simulink model "sim_PD_Control_wGC"  (R2020a)
settings: Solver=VariableStepAuto  StartTime=0.0  StopTime=T(end)  RelTol=1e-3
values from neighbouring files (symbols this model uses):
  q0 = zeros(1,NLinks)    [RobotPlot.m]
undefined symbols (not defined in the file or in its folder): B_accel, C_q, Fv_dq, fwdkin, G_q, Jadq, Jtrans, NLinks, T_step
settings Model: SimulationMode=accelerator  Creator=Dallas  LastModifiedBy=Dallas
settings DataIOCC: SaveFormat=Array  SaveOutput=off  SaveTime=off  ReturnWorkspaceOutputs=off

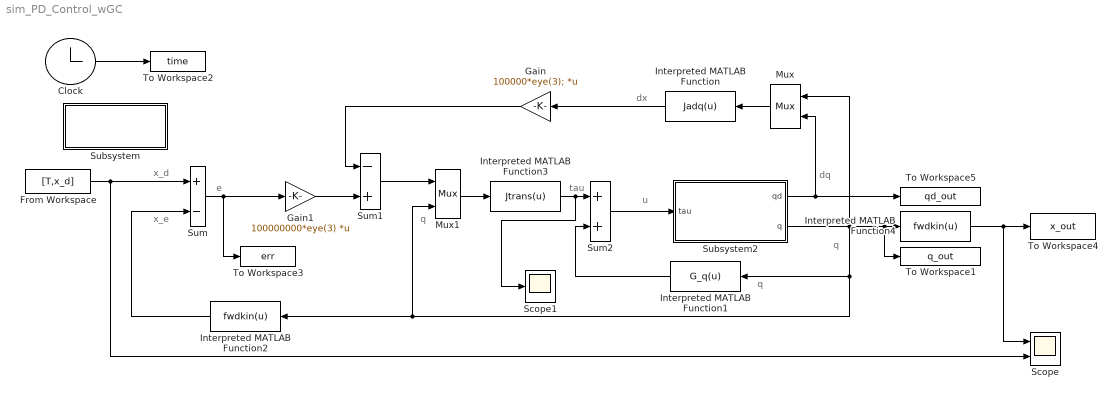
== system sim_PD_Control_wGC ==
  note: tau
  note: dx
  note: u
  note: q
  note: dq
  note: e
  note: x_e
  note: x_d
  note: q
  note: q
  Clock : Clock
  From Workspace : FromWorkspace  VariableName=[T,x_d]  SampleTime=T_step
  Gain : Gain  Gain=100000*eye(3);  Multiplication=Matrix(K*u)
      mask Display: disp('Kd')
  Gain1 : Gain  Gain=100000000*eye(3)  Multiplication=Matrix(K*u)
      mask Display: disp('Kp')
  Interpreted MATLAB Function : MATLABFcn  MATLABFcn=Jadq(u)  OutputDimensions=3
      mask Display: disp('Ja(q)*dq')
  Interpreted MATLAB Function1 : MATLABFcn  MATLABFcn=G_q(u)  OutputDimensions=NLinks
      mask Display: disp('G(q)')
  Interpreted MATLAB Function2 : MATLABFcn  MATLABFcn=fwdkin(u)  OutputDimensions=3
      mask Display: disp('Fwd Kin(q)')
  Interpreted MATLAB Function3 : MATLABFcn  MATLABFcn=Jtrans(u)  OutputDimensions=NLinks
      mask Display: disp('trans(Ja(dx))')
  Interpreted MATLAB Function4 : MATLABFcn  MATLABFcn=fwdkin(u)  OutputDimensions=3
      mask Display: disp('Fwd Kin(q)')
  Mux : Mux  Inputs=[NLinks,NLinks]
  Mux1 : Mux  Inputs=[3,NLinks]
  Scope : Scope  NumInputPorts=2
  Scope1 : Scope
  Subsystem : Subsystem  StartFcn=global NLinks DoF  StopFcn=SimPlotsPDG
      mask Display: disp('Plot')
  Subsystem2 : Subsystem
      mask Display: disp('inv(B(q))*(tau-tau'')')
  Sum : Sum  Inputs=+-
  Sum1 : Sum  Inputs=-+
  Sum2 : Sum
  To Workspace1 : ToWorkspace  VariableName=q_out  SampleTime=T_step
      settings: MaxDataPoints=4001
      mask Display: disp('q_out')
  To Workspace2 : ToWorkspace  VariableName=time  SampleTime=-1
      settings: MaxDataPoints=4001
      mask Display: disp('time')
  To Workspace3 : ToWorkspace  VariableName=err  SampleTime=T_step
      settings: MaxDataPoints=4001
      mask Display: disp('err')
  To Workspace4 : ToWorkspace  VariableName=x_out  SampleTime=T_step
      settings: MaxDataPoints=4001
      mask Display: disp('X_EEffector')
  To Workspace5 : ToWorkspace  VariableName=qd_out  SampleTime=T_step
      settings: MaxDataPoints=4001
      mask Display: disp('qd_out')
  wires:
  From Workspace/1 -> Scope/2, Sum/1
  Sum2/1 -> Subsystem2/1(tau)
  Subsystem2/1(qd) -> To Workspace5/1, Mux/2
  Subsystem2/2(q) -> To Workspace1/1, Interpreted MATLAB Function4/1, Mux1/2, Interpreted MATLAB Function2/1, Interpreted MATLAB Function1/1, Mux/1
  Interpreted MATLAB Function2/1 -> Sum/2
  Clock/1 -> To Workspace2/1
  Interpreted MATLAB Function1/1 -> Sum2/2
  Interpreted MATLAB Function3/1 -> Scope1/1, Sum2/1
  Mux/1 -> Interpreted MATLAB Function/1
  Mux1/1 -> Interpreted MATLAB Function3/1
  Interpreted MATLAB Function4/1 -> Scope/1, To Workspace4/1
  Sum/1 -> Gain1/1, To Workspace3/1
  Interpreted MATLAB Function/1 -> Gain/1
  Gain/1 -> Sum1/1
  Sum1/1 -> Mux1/1
  Gain1/1 -> Sum1/2

== system sim_PD_Control_wGC/Subsystem ==

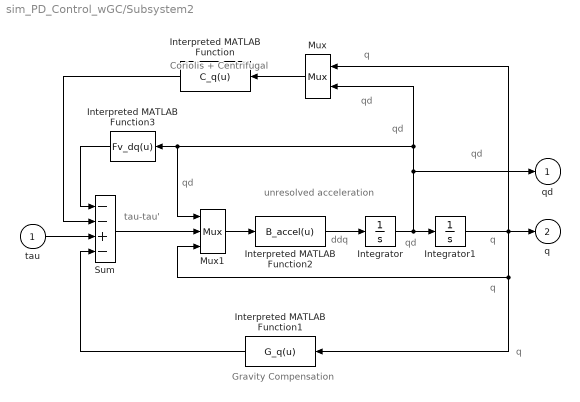
== system sim_PD_Control_wGC/Subsystem2 ==
  note: tau-tau'
  note: Gravity Compensation
  note: Coriolis + Centrifugal
  note: qd
  note: q
  note: unresolved
      | acceleration
  note: q
  note: q
  note: qd
  note: qd
  note: ddq
  note: q
  note: qd
  note: qd
  tau : Inport
  Integrator : Integrator
  Integrator1 : Integrator  InitialCondition=q0
  Interpreted MATLAB Function : MATLABFcn  MATLABFcn=C_q(u)  OutputDimensions=NLinks  Output1D=off
      mask Display: disp('C(q,dq)*dq')
  Interpreted MATLAB Function1 : MATLABFcn  MATLABFcn=G_q(u)  OutputDimensions=NLinks
      mask Display: disp('G(q)')
  Interpreted MATLAB Function2 : MATLABFcn  MATLABFcn=B_accel(u)  OutputDimensions=NLinks
      mask Display: disp('accel(q,dq,tau)')
  Interpreted MATLAB Function3 : MATLABFcn  MATLABFcn=Fv_dq(u)  OutputDimensions=NLinks
      mask Display: disp('Fv(dq)')
  Mux : Mux  Inputs=[NLinks,NLinks]
  Mux1 : Mux  Inputs=[NLinks,NLinks,NLinks]
  Sum : Sum  Inputs=--+-
  qd : Outport
  q : Outport  Port=2
  wires:
  tau/1 -> Sum/3
  Sum/1 -> Mux1/2
  Interpreted MATLAB Function2/1 -> Integrator/1
  Interpreted MATLAB Function1/1 -> Sum/4
  Integrator/1 -> Integrator1/1, Mux/2, Interpreted MATLAB Function3/1, Mux1/1, qd/1
  Interpreted MATLAB Function/1 -> Sum/2
  Interpreted MATLAB Function3/1 -> Sum/1
  Integrator1/1 -> Interpreted MATLAB Function1/1, Mux1/3, Mux/1, q/1
  Mux/1 -> Interpreted MATLAB Function/1
  Mux1/1 -> Interpreted MATLAB Function2/1
